simulink model "automata_learning"  (R2018a)
settings: Solver=VariableStepAuto  StartTime=0.0  StopTime=0.02  RelTol=1e-3
settings Model: Creator=xiaodong  LastModifiedBy=xiaodong

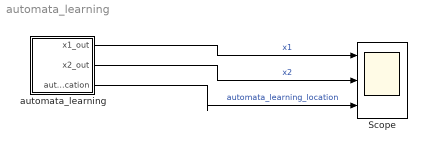
== system automata_learning ==
  Scope : Scope  NumInputPorts=3
  automata_learning : Stateflow chart  TreatAsAtomicUnit=on
  wires:
  automata_learning/1(x1_out) -> Scope/1  "x1"
  automata_learning/2(x2_out) -> Scope/2  "x2"
  automata_learning/3(automata_learning_location) -> Scope/3  "automata_learning_location"

== stateflow chart automata_learning/automata_learning ==
  settings: updateMethod=CONTINUOUS
  state loc2
    du:
    x1_dot = -78.31784197036177 * x1 - 150.3522015493363 * x2 - 1303.2842636667192;
    x2_dot = 181.73510726355016 * x1 - 17.66575048386585 * x2 - 606.3512578886002;
    x1_out=x1;
    x2_out=x2;
    automata_learning_location =2;
  state loc1
    du:
    x1_dot = 337004.9954586029 - 144.71542279189453 * x2 - 93.99660984519869 * x1;
    x2_dot = 181.94564409926534 * x1 - 18.128851790213957 * x2 - 131.46943390602246;
    x1_out=x1;
    x2_out=x2;
    automata_learning_location =1;
  state loc3
    du:
    x1_dot = 337004.9954586029 - 144.71542279189453 * x2 - 93.99660984519869 * x1;
    x2_dot = 181.94564409926534 * x1 - 18.128851790213957 * x2 - 131.46943390602246;
    x1_out=x1;
    x2_out=x2;
    automata_learning_location =3;
  state loc4
    du:
    x1_dot = 0.9974889665554656 * x1 - 0.09663260546039965 * x2 - 1.0;
    x2_dot = 0.008504421927369776 * x1 + 0.9719092445429851 * x2 - 1.0;
    x1_out=x1;
    x2_out=x2;
    automata_learning_location =4;
  loc1 -> loc2 : [0.000002948 * x1 - 0.0006628 * x2 + 1.0 < 0.0]
  loc3 -> loc4 : [-0.001953 * x1 - 0.0002316 * x2 + 1.0 > 0.0]
  (default) -> loc1 : {x1 = 0.0;
      | x2 = 0.0;}
  loc2 -> loc1 : [-0.0006627 * x2 + 1.0 > 0.0]
  data: x1_out output; x1 local; x2_out output; x2 local; automata_learning_location output
  data x1 settings: updateMethod=SF_CONTINUOUS_TIME_DATA
  data x2 settings: updateMethod=SF_CONTINUOUS_TIME_DATA
